simulink model "PubIfDecisionTOS_MDL"  (R2020b)
settings: configuration reference "DspaceConfig" (kept outside this file)
PostLoadFcn:
  | if any(exist('dsrtsu_mdlpostloadfcn', 'file') ~= 0), dsrtsu_mdlpostloadfcn('Execute', bdroot); end
InitFcn:
  | , if any(exist('dsmpb_private', 'file') ~= 0), dsmpb_private('dsmpb_mdlclblib', 'Init', bdroot); end,
undefined symbols (not defined in the file or in its folder): C_TOS_ACCEgoRAxletoFbumplength_m, C_TOS_ACCTargetFront_Flag, C_TOS_AEBJAPedObjDxThre_Val, C_TOS_AEBJAPedObjDyThre_Val, C_TOS_AEBJATargetSize_Val, C_TOS_AEBJAVehObjDxThre_Val, C_TOS_AEBJAVehObjDyThre_Val, C_TOS_AEBJuncPedTargetSize_Val, C_TOS_AEBLatObjDxThre_Val, C_TOS_AEBLatPedDyThre_Val, C_TOS_AEBLatTargetSize_Val, C_TOS_AEBLongTargetInEgoFront_Flag, C_TOS_axAbsGround_Parameter, C_TOS_CameraConfirmedFlag, C_TOS_CNsubjWidth, C_TOS_CurrentLaneCoreMinWidth_Val, C_TOS_CutInProb_Val_Zero, C_TOS_CutOutProb_Val_Zero, C_TOS_D2R_Val, C_TOS_DefaultValueObjectToCenterLine_dy, C_TOS_EgoCarWidth_Val, C_TOS_EgoDxRefPoint_m, C_TOS_EgoRAxletoFbumplength_m, C_TOS_HalfWidthVehicle_Con, C_TOS_HWA_CurrentLaneFlag, C_TOS_HWA_LeftLaneFlag, C_TOS_HWA_MovingDir_Vaild, C_TOS_HWA_MovState_Vaild, C_TOS_HWA_RightLaneFlag, C_TOS_LaneLineCourseErrorFront, C_TOS_LaneLineCourseErrorRear, C_TOS_MotorbikeDefaultWidth_m, C_TOS_NumberOfEffectiveTargets, C_TOS_Obj_Age_Val, C_TOS_Objdx_Constraint_Val, C_TOS_ObjectDefaultWidth_m, C_TOS_ObjInCurrentLane_Val, C_TOS_ObjInCurrentLaneValid, C_TOS_ObjInLeftLaneValid, C_TOS_ObjInRightLaneValid, C_TOS_ObjNotInCurrentLane_Val, C_TOS_ObjNotREElementType, C_TOS_ObjPredictDis_dy_ConstantVal_Zeros, C_TOS_ObjToCenterLine_ConstantVal_Zeros, C_TOS_OFMObjIDInvilad_Val, C_TOS_PIL_LatDisCons_Val_zero, C_TOS_PIL_ObjectCutInFlag_b, C_TOS_PIL_ObjectCutOutFlag_b, C_TOS_PIL_ObjLaneProb_al_Val, C_TOS_PP_ObjFusType_FC_Confirm_b, C_TOS_PP_ObjFusType_FC_FR_Confirm_b, C_TOS_PP_ObjFusType_FR_Confirm_b, C_TOS_RE_80BoolDefault_Val, C_TOS_RE_80Single181Default_Val, C_TOS_RE_80Single255Default_Val, C_TOS_RE_80Uint8Default_Val, C_TOS_RE_D2R, C_TOS_RE_D_180_Val, C_TOS_RE_InvalidObjectID_Val, C_TOS_RE_InvalidTargetChainDir_Val ... (+142)
libraries: simulink x1650, TOS_LIB x361, canfdmsglib x14
(part 28 of 69)

== system PubIfDecisionTOS_MDL/TOS_20201112/TOS_2012080320/TOS/ACC/TOS_ACCRightLane/ACC_LeftLane_Target/TOS_ACC_P3/ACC_P3_Targe ==
  ACC_P3_Index : Inport
  Object_Fus_Type : Inport  Port=2
  object_MovingState : Inport  Port=3
  PP_ObjMovingDirSignalProcessing : Inport  Port=4
  Object_HeadingAngle : Inport  Port=5
  Object_DX : Inport  Port=6
  Object_Type : Inport  Port=7
  Object_ObstacleProb : Inport  Port=8
  Object_DY : Inport  Port=9
  PP_ObjFusType_FC_FR_Confirm : Inport  Port=10
  PP_ObjFusType_FR_Confirm : Inport  Port=11
  PP_ObjFusType_FC_Confirm : Inport  Port=12
  Object_VX : Inport  Port=13
  Object_VY : Inport  Port=14
  VIE_EgoVelocity : Inport  Port=15
  SteerWheelAng : Inport  Port=16
  ACC_Target_ID_K1 : Inport  Port=17
  ACC_Target_ID_K2 : Inport  Port=18
  ACC_Target_MovState_K1 : Inport  Port=19
  ACC_Target_MovState_K2 : Inport  Port=20
  ObjectID : Inport  Port=21
  Action Port : ActionPort  ActionPortLabel=else
  ACC_P3_Targe : Subsystem
  Selector{1..3,5..13,15..16} (14 alike) : Selector  InputPortWidth=80  IndexOptions=Index vector (port)  Indices=[1 3]  OutputSizes=1
  ACC_P3_TargeConfirm : Outport
  TOS_ACC_FusionType_ObserVale : Outport  Port=2
  TOS_ACC_TrgMovDir_ObserVale : Outport  Port=3
  TOS_ACC_TargetDxConfirm_ObserVale : Outport  Port=4
  TOS_ACC_ObjType_ObserVale : Outport  Port=5
  TOS_ACC_ObstacleProb_ObserVale : Outport  Port=6
  TOS_ACC_TrgMovDirFlag_1_ObserVale : Outport  Port=7
  TOS_ACC_TrgMovDirFlag_2_ObserVale : Outport  Port=8
  TOS_ACC_TrgMovDirFlag_3_ObserVale : Outport  Port=9
  TOS_ACC_TrgMovDirFlag_4_ObserVale : Outport  Port=10
  TOS_ACC_TrgMovDirFlag_5_ObserVale : Outport  Port=11
  TOS_ACC_TrgMovDirFlag_6_ObserVale : Outport  Port=12
  wires:
  ACC_P3_Targe/12(TOS_ACC_TrgMovDirFlag_6_ObserVale) -> TOS_ACC_TrgMovDirFlag_6_ObserVale/1
  ACC_P3_Targe/11(TOS_ACC_TrgMovDirFlag_5_ObserVale) -> TOS_ACC_TrgMovDirFlag_5_ObserVale/1
  ACC_P3_Targe/1(ACC_P3_TargeConfirm) -> ACC_P3_TargeConfirm/1
  ACC_P3_Targe/10(TOS_ACC_TrgMovDirFlag_4_ObserVale) -> TOS_ACC_TrgMovDirFlag_4_ObserVale/1
  ACC_P3_Targe/2(TOS_ACC_FusionType_ObserVale) -> TOS_ACC_FusionType_ObserVale/1
  ACC_P3_Targe/9(TOS_ACC_TrgMovDirFlag_3_ObserVale) -> TOS_ACC_TrgMovDirFlag_3_ObserVale/1
  ACC_P3_Targe/3(TOS_ACC_TrgMovDir_ObserVale) -> TOS_ACC_TrgMovDir_ObserVale/1
  ACC_P3_Targe/8(TOS_ACC_TrgMovDirFlag_2_ObserVale) -> TOS_ACC_TrgMovDirFlag_2_ObserVale/1
  ACC_P3_Targe/4(TOS_ACC_TargetDxConfirm_ObserVale) -> TOS_ACC_TargetDxConfirm_ObserVale/1
  ACC_P3_Targe/7(TOS_ACC_TrgMovDirFlag_1_ObserVale) -> TOS_ACC_TrgMovDirFlag_1_ObserVale/1
  ACC_P3_Targe/5(TOS_ACC_ObjType_ObserVale) -> TOS_ACC_ObjType_ObserVale/1
  ACC_P3_Targe/6(TOS_ACC_ObstacleProb_ObserVale) -> TOS_ACC_ObstacleProb_ObserVale/1
  ACC_P3_Index/1 -> Selector16/2, Selector3/2, Selector2/2, Selector5/2, Selector6/2, Selector7/2, Selector8/2, Selector9/2, Selector10/2, Selector11/2, Selector15/2, Selector12/2, Selector13/2, Selector1/2
  Selector3/1 -> ACC_P3_Targe/20(ObjectID)
  Selector2/1 -> ACC_P3_Targe/13(Object_VY)
  Selector5/1 -> ACC_P3_Targe/12(Object_VX)
  Selector6/1 -> ACC_P3_Targe/11(PP_ObjFusType_FC_Confirm)
  Selector7/1 -> ACC_P3_Targe/10(PP_ObjFusType_FR_Confirm)
  Selector8/1 -> ACC_P3_Targe/9(PP_ObjFusType_FC_FR_Confirm)
  Selector9/1 -> ACC_P3_Targe/8(Object_DY)
  Selector10/1 -> ACC_P3_Targe/7(Object_ObstacleProb)
  Selector11/1 -> ACC_P3_Targe/6(Object_Type)
  Selector15/1 -> ACC_P3_Targe/5(Object_DX)
  Selector16/1 -> ACC_P3_Targe/4(Object_HeadingAngle)
  Selector12/1 -> ACC_P3_Targe/3(PP_ObjMovingDirSignalProcessing)
  Selector13/1 -> ACC_P3_Targe/2(object_MovingState)
  Selector1/1 -> ACC_P3_Targe/1(Object_Fus_Type)
  ObjectID/1 -> Selector3/1
  ACC_Target_MovState_K2/1 -> ACC_P3_Targe/19(ACC_Target_MovState_K2)
  ACC_Target_MovState_K1/1 -> ACC_P3_Targe/18(ACC_Target_MovState_K1)
  ACC_Target_ID_K2/1 -> ACC_P3_Targe/17(ACC_Target_ID_K2)
  ACC_Target_ID_K1/1 -> ACC_P3_Targe/16(ACC_Target_ID_K1)
  SteerWheelAng/1 -> ACC_P3_Targe/15(SteerWheelAng)
  VIE_EgoVelocity/1 -> ACC_P3_Targe/14(VIE_EgoVelocity)
  Object_VY/1 -> Selector2/1
  Object_VX/1 -> Selector5/1
  PP_ObjFusType_FC_Confirm/1 -> Selector6/1
  PP_ObjFusType_FR_Confirm/1 -> Selector7/1
  PP_ObjFusType_FC_FR_Confirm/1 -> Selector8/1
  Object_DY/1 -> Selector9/1
  Object_ObstacleProb/1 -> Selector10/1
  Object_Type/1 -> Selector11/1
  Object_DX/1 -> Selector15/1
  Object_HeadingAngle/1 -> Selector16/1
  PP_ObjMovingDirSignalProcessing/1 -> Selector12/1
  object_MovingState/1 -> Selector13/1
  Object_Fus_Type/1 -> Selector1/1

== system PubIfDecisionTOS_MDL/TOS_20201112/TOS_2012080320/TOS/ACC/TOS_ACCRightLane/ACC_LeftLane_Target/TOS_ACC_P3/ACC_P3_TargeDefault ==
  Action Port : ActionPort  ActionPortLabel=if(u1 ~= 0)
  Constant{1..6,8..13} (12 alike) : Constant  Value=0  OutDataTypeStr=boolean
  ACC_P3_TargeConfirm : Outport
  TOS_ACC_FusionType_ObserVale : Outport  Port=2
  TOS_ACC_TrgMovDir_ObserVale : Outport  Port=3
  TOS_ACC_TargetDxConfirm_ObserVale : Outport  Port=4
  TOS_ACC_ObjType_ObserVale : Outport  Port=5
  TOS_ACC_ObstacleProb_ObserVale : Outport  Port=6
  TOS_ACC_TrgMovDirFlag_1_ObserVale : Outport  Port=7
  TOS_ACC_TrgMovDirFlag_2_ObserVale : Outport  Port=8
  TOS_ACC_TrgMovDirFlag_3_ObserVale : Outport  Port=9
  TOS_ACC_TrgMovDirFlag_4_ObserVale : Outport  Port=10
  TOS_ACC_TrgMovDirFlag_5_ObserVale : Outport  Port=11
  TOS_ACC_TrgMovDirFlag_6_ObserVale : Outport  Port=12
  wires:
  Constant13/1 -> TOS_ACC_TrgMovDirFlag_6_ObserVale/1
  Constant12/1 -> TOS_ACC_TrgMovDirFlag_5_ObserVale/1
  Constant11/1 -> TOS_ACC_TrgMovDirFlag_4_ObserVale/1
  Constant10/1 -> TOS_ACC_TrgMovDirFlag_3_ObserVale/1
  Constant9/1 -> TOS_ACC_TrgMovDirFlag_2_ObserVale/1
  Constant8/1 -> TOS_ACC_TrgMovDirFlag_1_ObserVale/1
  Constant6/1 -> TOS_ACC_ObstacleProb_ObserVale/1
  Constant5/1 -> TOS_ACC_ObjType_ObserVale/1
  Constant4/1 -> TOS_ACC_TargetDxConfirm_ObserVale/1
  Constant3/1 -> TOS_ACC_TrgMovDir_ObserVale/1
  Constant1/1 -> TOS_ACC_FusionType_ObserVale/1
  Constant2/1 -> ACC_P3_TargeConfirm/1

== system PubIfDecisionTOS_MDL/TOS_20201112/TOS_2012080320/TOS/ACC/TOS_ACCRightLane/ACC_LeftLane_Target/TOS_ACC_P5/ACC_P5_Targe ==
  ACC_P5_Index : Inport
  Object_Fus_Type : Inport  Port=2
  object_MovingState : Inport  Port=3
  PP_ObjMovingDirSignalProcessing : Inport  Port=4
  Object_HeadingAngle : Inport  Port=5
  Object_DX : Inport  Port=6
  Object_Type : Inport  Port=7
  Object_ObstacleProb : Inport  Port=8
  Object_DY : Inport  Port=9
  PP_ObjFusType_FC_FR_Confirm : Inport  Port=10
  PP_ObjFusType_FR_Confirm : Inport  Port=11
  PP_ObjFusType_FC_Confirm : Inport  Port=12
  Object_VX : Inport  Port=13
  Object_VY : Inport  Port=14
  VIE_EgoVelocity : Inport  Port=15
  SteerWheelAng : Inport  Port=16
  ACC_Target_ID_K1 : Inport  Port=17
  ACC_Target_ID_K2 : Inport  Port=18
  ACC_Target_MovState_K1 : Inport  Port=19
  ACC_Target_MovState_K2 : Inport  Port=20
  ObjectID : Inport  Port=21
  Action Port : ActionPort  ActionPortLabel=else
  ACC_P5_Targe : Subsystem
  Selector{1..3,5..13,15..16} (14 alike) : Selector  InputPortWidth=80  IndexOptions=Index vector (port)  Indices=[1 3]  OutputSizes=1
  ACC_P5_TargeConfirm : Outport
  TOS_ACC_FusionType_ObserVale : Outport  Port=2
  TOS_ACC_TrgMovDir_ObserVale : Outport  Port=3
  TOS_ACC_TargetDxConfirm_ObserVale : Outport  Port=4
  TOS_ACC_ObjType_ObserVale : Outport  Port=5
  TOS_ACC_ObstacleProb_ObserVale : Outport  Port=6
  TOS_ACC_TrgMovDirFlag_1_ObserVale : Outport  Port=7
  TOS_ACC_TrgMovDirFlag_2_ObserVale : Outport  Port=8
  TOS_ACC_TrgMovDirFlag_3_ObserVale : Outport  Port=9
  TOS_ACC_TrgMovDirFlag_4_ObserVale : Outport  Port=10
  TOS_ACC_TrgMovDirFlag_5_ObserVale : Outport  Port=11
  TOS_ACC_TrgMovDirFlag_6_ObserVale : Outport  Port=12
  wires:
  Object_Fus_Type/1 -> Selector1/1
  object_MovingState/1 -> Selector13/1
  PP_ObjMovingDirSignalProcessing/1 -> Selector12/1
  Object_HeadingAngle/1 -> Selector16/1
  Object_DX/1 -> Selector15/1
  Object_Type/1 -> Selector11/1
  Object_ObstacleProb/1 -> Selector10/1
  Object_DY/1 -> Selector9/1
  PP_ObjFusType_FC_FR_Confirm/1 -> Selector8/1
  PP_ObjFusType_FR_Confirm/1 -> Selector7/1
  PP_ObjFusType_FC_Confirm/1 -> Selector6/1
  Object_VX/1 -> Selector5/1
  Object_VY/1 -> Selector2/1
  VIE_EgoVelocity/1 -> ACC_P5_Targe/14(VIE_EgoVelocity)
  SteerWheelAng/1 -> ACC_P5_Targe/15(SteerWheelAng)
  ACC_Target_ID_K1/1 -> ACC_P5_Targe/16(ACC_Target_ID_K1)
  ACC_Target_ID_K2/1 -> ACC_P5_Targe/17(ACC_Target_ID_K2)
  ACC_Target_MovState_K1/1 -> ACC_P5_Targe/18(ACC_Target_MovState_K1)
  ACC_Target_MovState_K2/1 -> ACC_P5_Targe/19(ACC_Target_MovState_K2)
  ObjectID/1 -> Selector3/1
  Selector1/1 -> ACC_P5_Targe/1(Object_Fus_Type)
  Selector13/1 -> ACC_P5_Targe/2(object_MovingState)
  Selector12/1 -> ACC_P5_Targe/3(PP_ObjMovingDirSignalProcessing)
  Selector16/1 -> ACC_P5_Targe/4(Object_HeadingAngle)
  Selector15/1 -> ACC_P5_Targe/5(Object_DX)
  Selector11/1 -> ACC_P5_Targe/6(Object_Type)
  Selector10/1 -> ACC_P5_Targe/7(Object_ObstacleProb)
  Selector9/1 -> ACC_P5_Targe/8(Object_DY)
  Selector8/1 -> ACC_P5_Targe/9(PP_ObjFusType_FC_FR_Confirm)
  Selector7/1 -> ACC_P5_Targe/10(PP_ObjFusType_FR_Confirm)
  Selector6/1 -> ACC_P5_Targe/11(PP_ObjFusType_FC_Confirm)
  Selector5/1 -> ACC_P5_Targe/12(Object_VX)
  Selector2/1 -> ACC_P5_Targe/13(Object_VY)
  Selector3/1 -> ACC_P5_Targe/20(ObjectID)
  ACC_P5_Index/1 -> Selector1/2, Selector13/2, Selector12/2, Selector15/2, Selector11/2, Selector10/2, Selector9/2, Selector8/2, Selector7/2, Selector6/2, Selector5/2, Selector2/2, Selector3/2, Selector16/2
  ACC_P5_Targe/6(TOS_ACC_ObstacleProb_ObserVale) -> TOS_ACC_ObstacleProb_ObserVale/1
  ACC_P5_Targe/5(TOS_ACC_ObjType_ObserVale) -> TOS_ACC_ObjType_ObserVale/1
  ACC_P5_Targe/7(TOS_ACC_TrgMovDirFlag_1_ObserVale) -> TOS_ACC_TrgMovDirFlag_1_ObserVale/1
  ACC_P5_Targe/4(TOS_ACC_TargetDxConfirm_ObserVale) -> TOS_ACC_TargetDxConfirm_ObserVale/1
  ACC_P5_Targe/8(TOS_ACC_TrgMovDirFlag_2_ObserVale) -> TOS_ACC_TrgMovDirFlag_2_ObserVale/1
  ACC_P5_Targe/3(TOS_ACC_TrgMovDir_ObserVale) -> TOS_ACC_TrgMovDir_ObserVale/1
  ACC_P5_Targe/9(TOS_ACC_TrgMovDirFlag_3_ObserVale) -> TOS_ACC_TrgMovDirFlag_3_ObserVale/1
  ACC_P5_Targe/2(TOS_ACC_FusionType_ObserVale) -> TOS_ACC_FusionType_ObserVale/1
  ACC_P5_Targe/10(TOS_ACC_TrgMovDirFlag_4_ObserVale) -> TOS_ACC_TrgMovDirFlag_4_ObserVale/1
  ACC_P5_Targe/1(ACC_P5_TargeConfirm) -> ACC_P5_TargeConfirm/1
  ACC_P5_Targe/11(TOS_ACC_TrgMovDirFlag_5_ObserVale) -> TOS_ACC_TrgMovDirFlag_5_ObserVale/1
  ACC_P5_Targe/12(TOS_ACC_TrgMovDirFlag_6_ObserVale) -> TOS_ACC_TrgMovDirFlag_6_ObserVale/1

== system PubIfDecisionTOS_MDL/TOS_20201112/TOS_2012080320/TOS/ACC/TOS_ACCRightLane/ACC_LeftLane_Target/TOS_ACC_P5/ACC_P5_TargeDefault ==
  Action Port : ActionPort  ActionPortLabel=if(u1 ~= 0)
  Constant{1..6,8..13} (12 alike) : Constant  Value=0  OutDataTypeStr=boolean
  ACC_P5_TargeConfirm : Outport
  TOS_ACC_FusionType_ObserVale : Outport  Port=2
  TOS_ACC_TrgMovDir_ObserVale : Outport  Port=3
  TOS_ACC_TargetDxConfirm_ObserVale : Outport  Port=4
  TOS_ACC_ObjType_ObserVale : Outport  Port=5
  TOS_ACC_ObstacleProb_ObserVale : Outport  Port=6
  TOS_ACC_TrgMovDirFlag_1_ObserVale : Outport  Port=7
  TOS_ACC_TrgMovDirFlag_2_ObserVale : Outport  Port=8
  TOS_ACC_TrgMovDirFlag_3_ObserVale : Outport  Port=9
  TOS_ACC_TrgMovDirFlag_4_ObserVale : Outport  Port=10
  TOS_ACC_TrgMovDirFlag_5_ObserVale : Outport  Port=11
  TOS_ACC_TrgMovDirFlag_6_ObserVale : Outport  Port=12
  wires:
  Constant2/1 -> ACC_P5_TargeConfirm/1
  Constant1/1 -> TOS_ACC_FusionType_ObserVale/1
  Constant3/1 -> TOS_ACC_TrgMovDir_ObserVale/1
  Constant4/1 -> TOS_ACC_TargetDxConfirm_ObserVale/1
  Constant5/1 -> TOS_ACC_ObjType_ObserVale/1
  Constant6/1 -> TOS_ACC_ObstacleProb_ObserVale/1
  Constant8/1 -> TOS_ACC_TrgMovDirFlag_1_ObserVale/1
  Constant9/1 -> TOS_ACC_TrgMovDirFlag_2_ObserVale/1
  Constant10/1 -> TOS_ACC_TrgMovDirFlag_3_ObserVale/1
  Constant11/1 -> TOS_ACC_TrgMovDirFlag_4_ObserVale/1
  Constant12/1 -> TOS_ACC_TrgMovDirFlag_5_ObserVale/1
  Constant13/1 -> TOS_ACC_TrgMovDirFlag_6_ObserVale/1

== system PubIfDecisionTOS_MDL/TOS_20201112/TOS_2012080320/TOS/ACC/TOS_ACCRightLane/ACC_Object_PreConfirm/ACC_Object_PreConfirm/ACC_Object_PreConfirm ==
  Object_ID : Inport
  PP_ObjFusType_FC_FR_Confirm : Inport  Port=2
  PP_ObjFusType_FR_Confirm : Inport  Port=3
  PP_ObjFusType_FC_Confirm : Inport  Port=4
  Obj_MovingState : Inport  Port=5
  Obj_Dx : Inport  Port=6
  Object_ObstacleProb : Inport  Port=7
  Object_DY : Inport  Port=8
  Object_ObjType : Inport  Port=9
  ACC_Target_ID_K1 : Inport  Port=10
  ACC_Target_Dx_K1 : Inport  Port=11
  Action Port : ActionPort  ActionPortLabel=else
  " " : Subsystem
  Bus Creator : BusCreator  Inputs=11
  Bus Selector1 : BusSelector  OutputSignals=PP_ObjFusType_FC_Confirm,Obj_MovingState
  Bus Selector2 : BusSelector  OutputSignals=PP_ObjFusType_FC_FR_Confirm,PP_ObjFusType_FC_Confirm,PP_ObjFusType_FR_Confirm
  Bus Selector4 : BusSelector  OutputSignals=Object_ObjType
  Constant1 : Constant  OutDataTypeStr=boolean
  Logical Operator1 : Logic  Inputs=4  AllPortsSameDT=off  OutDataTypeStr=boolean
  Subsystem : Subsystem
  Subsystem1 : Subsystem
  TOS_ACC_DyConfirm : Subsystem
  Terminator : Terminator
  TOS_ACC_TargetPre_Confirm_FiltFlag : Outport
  TOS_ACC_TargetPre_FusionTypeFlag_ObserVale : Outport  Port=2
  TOS_ACC_TargetPre_PassedbyTarget_ObserVale : Outport  Port=3
  TOS_ACC_TargetPre_ObjType_ObserVale : Outport  Port=4
  TOS_ACC_DyConfirm_ObserVale : Outport  Port=5
  wires:
  TOS_ACC_DyConfirm/1(TOS_ACC_TargetPre_DyConfirm) -> Terminator/1
  Bus Creator/1 -> Bus Selector2/1, Bus Selector1/1, Bus Selector4/1, TOS_ACC_DyConfirm/1(TOS_ACC_Dy)
  Logical Operator1/1 -> TOS_ACC_TargetPre_Confirm_FiltFlag/1
  [TOS_ACC_DyConfirm_ObserVale] -> TOS_ACC_DyConfirm_ObserVale/1
  Constant1/1 -> [TOS_ACC_DyConfirm_ObserVale], Logical Operator1/4
  [TOS_ACC_TargetPre_ObjType_ObserVale] -> TOS_ACC_TargetPre_ObjType_ObserVale/1
  [TOS_ACC_TargetPre_PassedbyTarget_Flag_ObserVale] -> TOS_ACC_TargetPre_PassedbyTarget_ObserVale/1
  [TOS_ACC_TargetPre_FusionTypeFlag_ObserVale] -> TOS_ACC_TargetPre_FusionTypeFlag_ObserVale/1
  Object_ObjType/1 -> Bus Creator/9  "Object_ObjType"
  " "/1(TOS_ACC_TargetPre_ObjType) -> [TOS_ACC_TargetPre_ObjType_ObserVale], Logical Operator1/3
  Bus Selector4/1 -> " "/1(Object_Type)  "<Object_ObjType>"
  Obj_Dx/1 -> Bus Creator/6  "Obj_Dx"
  Object_ObstacleProb/1 -> Bus Creator/7  "Object_ObstacleProb"
  Obj_MovingState/1 -> Bus Creator/5  "Obj_MovingState"
  ACC_Target_Dx_K1/1 -> Bus Creator/11  "ACC_Target_Dx_K1"
  Bus Selector1/2 -> Subsystem1/2(Obj_MovingState)  "<Obj_MovingState>"
  Object_DY/1 -> Bus Creator/8  "Object_DY"
  ACC_Target_ID_K1/1 -> Bus Creator/10  "ACC_Target_ID_K1"
  PP_ObjFusType_FC_FR_Confirm/1 -> Bus Creator/2  "PP_ObjFusType_FC_FR_Confirm"
  Bus Selector2/2 -> Subsystem/2(PP_ObjFusType_FR_Confirm)  "<PP_ObjFusType_FC_Confirm>"
  Bus Selector1/1 -> Subsystem1/1(PP_ObjFusType_FC_Confirm)  "<PP_ObjFusType_FC_Confirm>"
  Bus Selector2/3 -> Subsystem/3(PP_ObjFusType_FC_Confirm)  "<PP_ObjFusType_FR_Confirm>"
  Bus Selector2/1 -> Subsystem/1(PP_ObjFusType_FC_FR_Confirm)  "<PP_ObjFusType_FC_FR_Confirm>"
  PP_ObjFusType_FC_Confirm/1 -> Bus Creator/4  "PP_ObjFusType_FC_Confirm"
  Object_ID/1 -> Bus Creator/1  "Object_ID"
  PP_ObjFusType_FR_Confirm/1 -> Bus Creator/3  "PP_ObjFusType_FR_Confirm"
  Subsystem1/1(TOS_ACC_TargetPre_ObjectPassedbyTarget_Flag) -> Logical Operator1/2, [TOS_ACC_TargetPre_PassedbyTarget_Flag_ObserVale]
  Subsystem/1(TOS_ACC_TargetPre_TargetFusionTypeFlag) -> Logical Operator1/1, [TOS_ACC_TargetPre_FusionTypeFlag_ObserVale]

== system PubIfDecisionTOS_MDL/TOS_20201112/TOS_2012080320/TOS/ACC/TOS_ACCRightLane/ACC_Object_PreConfirm/ACC_Object_PreConfirm/ACC_Object_PreConfirmDefault ==
  Action Port : ActionPort  ActionPortLabel=if(u1 ~= 0)
  Constant{2,5..6,8,10} (5 alike) : Constant  Value=0  OutDataTypeStr=boolean
  TOS_ACC_TargetPre_Confirm_FiltFlag : Outport
  TOS_ACC_TargetPre_FusionTypeFlag_ObserVale : Outport  Port=2
  TOS_ACC_TargetPre_PassedbyTarget_ObserVale : Outport  Port=3
  TOS_ACC_TargetPre_ObjType_ObserVale : Outport  Port=4
  TOS_ACC_DyConfirm_ObserVale : Outport  Port=5
  wires:
  Constant10/1 -> TOS_ACC_DyConfirm_ObserVale/1
  Constant8/1 -> TOS_ACC_TargetPre_ObjType_ObserVale/1
  Constant6/1 -> TOS_ACC_TargetPre_PassedbyTarget_ObserVale/1
  Constant5/1 -> TOS_ACC_TargetPre_FusionTypeFlag_ObserVale/1
  Constant2/1 -> TOS_ACC_TargetPre_Confirm_FiltFlag/1

== system PubIfDecisionTOS_MDL/TOS_20201112/TOS_2012080320/TOS/AEB/TOS_AEBJunct1105/AEBJunc_Object_Condition/AEBJA_TargetCondition/TOS_AEBJunc_TargetsCondition ==
  Object_ID : Inport
  PP_ObjFusType_FC_FR_Confirm : Inport  Port=2
  PP_ObjFusType_FR_Confirm : Inport  Port=3
  ObjectType : Inport  Port=4
  Object_Dx : Inport  Port=5
  Object_Dy : Inport  Port=6
  PP_ObjMovingDirSignalProcessing : Inport  Port=7
  Object_HeadingAngle : Inport  Port=8
  Object_VX : Inport  Port=9
  Object_VY : Inport  Port=10
  VIE_EgoVelocity : Inport  Port=11
  psiDtOpt : Inport  Port=12
  axvRefMs2 : Inport  Port=13
  Object_MovingState : Inport  Port=14
  AEBJunc_Target_ObjectID_K1 : Inport  Port=15
  AEBJunc_Target_ObjectType_K1 : Inport  Port=16
  Action Port : ActionPort
  AEBJunc_PedTargetCondition : Subsystem
  AEBJunc_VehTargetCondition : Subsystem
  Bus Creator : BusCreator  Inputs=16
  Bus Selector : BusSelector  OutputSignals=Object_ID,PP_ObjFusType_FC_FR_Confirm,PP_ObjFusType_FR_Confirm,ObjectType,Object_Dx,Object_Dy,PP_ObjMovingDirSignalProcessing,Object_HeadingAngle,Object_VX,Object_VY,VIE_EgoVelocity,psiDtOpt,axvRefMs2,AEBJunc_Target_ObjectID_K1,AEBJunc_Target_ObjectType_K1
  Bus Selector1 : BusSelector  OutputSignals=Object_ID,PP_ObjFusType_FC_FR_Confirm,PP_ObjFusType_FR_Confirm,ObjectType,Object_Dx,Object_Dy,PP_ObjMovingDirSignalProcessing,Object_HeadingAngle,Object_VX,Object_VY,VIE_EgoVelocity,psiDtOpt,axvRefMs2,AEBJunc_Target_ObjectID_K1,AEBJunc_Target_ObjectType_K1,Object_MovingState
  TOS_AEBJunc_PedTargetsDx : Outport
  TOS_AEBJunc_VehTargetsDx : Outport  Port=2
  AEBJunc_PedTargetFusionType_observal : Outport  Port=3
  AEBJunc_PedTargetObjectType_observal : Outport  Port=4
  AEBJunc_PedTargetDXDY_observal : Outport  Port=5
  AEBJunc_PedTargetMovDir_observal : Outport  Port=6
  AEBJunc_VehTargetFusionType_observal : Outport  Port=7
  AEBJunc_VehTargetObjectType_observal : Outport  Port=8
  AEBJunc_VehTargetDXDY_observal : Outport  Port=9
  AEBJunc_VehTargetMovDir_observal : Outport  Port=10
  AEBJunc_VehTargetMovState_observal : Outport  Port=11
  wires:
  AEBJunc_PedTargetCondition/1(TOS_AEBJunc_PedTargetsDx) -> TOS_AEBJunc_PedTargetsDx/1
  AEBJunc_PedTargetCondition/2(AEBJunc_PedTargetFusionType_observal) -> AEBJunc_PedTargetFusionType_observal/1
  AEBJunc_PedTargetCondition/3(AEBJunc_PedTargetObjectType_observal) -> AEBJunc_PedTargetObjectType_observal/1
  AEBJunc_PedTargetCondition/4(AEBJunc_PedTargetDXDY_observal) -> AEBJunc_PedTargetDXDY_observal/1
  AEBJunc_PedTargetCondition/5(AEBJunc_PedTargetMovDir_observal) -> AEBJunc_PedTargetMovDir_observal/1
  Object_ID/1 -> Bus Creator/1  "Object_ID"
  PP_ObjFusType_FC_FR_Confirm/1 -> Bus Creator/2  "PP_ObjFusType_FC_FR_Confirm"
  PP_ObjFusType_FR_Confirm/1 -> Bus Creator/3  "PP_ObjFusType_FR_Confirm"
  ObjectType/1 -> Bus Creator/4  "ObjectType"
  Object_Dx/1 -> Bus Creator/5  "Object_Dx"
  Object_Dy/1 -> Bus Creator/6  "Object_Dy"
  PP_ObjMovingDirSignalProcessing/1 -> Bus Creator/7  "PP_ObjMovingDirSignalProcessing"
  Object_HeadingAngle/1 -> Bus Creator/8  "Object_HeadingAngle"
  Object_VX/1 -> Bus Creator/9  "Object_VX"
  Object_VY/1 -> Bus Creator/10  "Object_VY"
  VIE_EgoVelocity/1 -> Bus Creator/11  "VIE_EgoVelocity"
  psiDtOpt/1 -> Bus Creator/12  "psiDtOpt"
  axvRefMs2/1 -> Bus Creator/13  "axvRefMs2"
  AEBJunc_Target_ObjectID_K1/1 -> Bus Creator/15  "AEBJunc_Target_ObjectID_K1"
  AEBJunc_Target_ObjectType_K1/1 -> Bus Creator/16  "AEBJunc_Target_ObjectType_K1"
  Bus Creator/1 -> Bus Selector1/1, Bus Selector/1
  Bus Selector/1 -> AEBJunc_PedTargetCondition/1(Object_ID)  "<Object_ID>"
  Bus Selector/2 -> AEBJunc_PedTargetCondition/2(PP_ObjFusType_FC_FR_Confirm)  "<PP_ObjFusType_FC_FR_Confirm>"
  Bus Selector/3 -> AEBJunc_PedTargetCondition/3(PP_ObjFusType_FR_Confirm)  "<PP_ObjFusType_FR_Confirm>"
  Bus Selector/4 -> AEBJunc_PedTargetCondition/4(ObjectType)  "<ObjectType>"
  Bus Selector/5 -> AEBJunc_PedTargetCondition/5(Object_Dx)  "<Object_Dx>"
  Bus Selector/6 -> AEBJunc_PedTargetCondition/6(Object_Dy)  "<Object_Dy>"
  Bus Selector/7 -> AEBJunc_PedTargetCondition/7(PP_ObjMovingDirSignalProcessing)  "<PP_ObjMovingDirSignalProcessing>"
  Bus Selector/8 -> AEBJunc_PedTargetCondition/8(Object_HeadingAngle)  "<Object_HeadingAngle>"
  Bus Selector/9 -> AEBJunc_PedTargetCondition/9(Object_VX)  "<Object_VX>"
  Bus Selector/10 -> AEBJunc_PedTargetCondition/10(Object_VY)  "<Object_VY>"
  Bus Selector/11 -> AEBJunc_PedTargetCondition/11(VIE_EgoVelocity)  "<VIE_EgoVelocity>"
  Bus Selector/12 -> AEBJunc_PedTargetCondition/12(psiDtOpt)  "<psiDtOpt>"
  Bus Selector/13 -> AEBJunc_PedTargetCondition/13(axvRefMs2)  "<axvRefMs2>"
  Bus Selector/14 -> AEBJunc_PedTargetCondition/14(AEBJunc_PedTarget_ObjectID_K1)  "<AEBJunc_Target_ObjectID_K1>"
  Bus Selector/15 -> AEBJunc_PedTargetCondition/15(AEBJunc_Target_ObjectType_K1)  "<AEBJunc_Target_ObjectType_K1>"
  Bus Selector1/15 -> AEBJunc_VehTargetCondition/15(AEBJunc_Target_ObjectType_K1)  "<AEBJunc_Target_ObjectType_K1>"
  Bus Selector1/14 -> AEBJunc_VehTargetCondition/14(AEBJunc_VehTarget_ObjectID_K1)  "<AEBJunc_Target_ObjectID_K1>"
  Bus Selector1/13 -> AEBJunc_VehTargetCondition/13(axvRefMs2)  "<axvRefMs2>"
  Bus Selector1/12 -> AEBJunc_VehTargetCondition/12(psiDtOpt)  "<psiDtOpt>"
  Bus Selector1/11 -> AEBJunc_VehTargetCondition/11(VIE_EgoVelocity)  "<VIE_EgoVelocity>"
  Bus Selector1/10 -> AEBJunc_VehTargetCondition/10(Object_VY)  "<Object_VY>"
  Bus Selector1/9 -> AEBJunc_VehTargetCondition/9(Object_VX)  "<Object_VX>"
  Bus Selector1/8 -> AEBJunc_VehTargetCondition/8(Object_HeadingAngle)  "<Object_HeadingAngle>"
  Bus Selector1/7 -> AEBJunc_VehTargetCondition/7(PP_ObjMovingDirSignalProcessing)  "<PP_ObjMovingDirSignalProcessing>"
  Bus Selector1/6 -> AEBJunc_VehTargetCondition/6(Object_Dy)  "<Object_Dy>"
  Bus Selector1/5 -> AEBJunc_VehTargetCondition/5(Object_Dx)  "<Object_Dx>"
  Bus Selector1/4 -> AEBJunc_VehTargetCondition/4(ObjectType)  "<ObjectType>"
  Bus Selector1/3 -> AEBJunc_VehTargetCondition/3(PP_ObjFusType_FR_Confirm)  "<PP_ObjFusType_FR_Confirm>"
  Bus Selector1/2 -> AEBJunc_VehTargetCondition/2(PP_ObjFusType_FC_FR_Confirm)  "<PP_ObjFusType_FC_FR_Confirm>"
  Bus Selector1/1 -> AEBJunc_VehTargetCondition/1(Object_ID)  "<Object_ID>"
  AEBJunc_VehTargetCondition/5(AEBJunc_VehTargetMovDir_observal) -> AEBJunc_VehTargetMovDir_observal/1
  AEBJunc_VehTargetCondition/4(AEBJunc_VehTargetDXDY_observal) -> AEBJunc_VehTargetDXDY_observal/1
  AEBJunc_VehTargetCondition/3(AEBJunc_VehTargetObjectType_observal) -> AEBJunc_VehTargetObjectType_observal/1
  AEBJunc_VehTargetCondition/2(AEBJunc_VehTargetFusionType_observal) -> AEBJunc_VehTargetFusionType_observal/1
  AEBJunc_VehTargetCondition/1(TOS_AEBJunc_VehTargetsDx) -> TOS_AEBJunc_VehTargetsDx/1
  Object_MovingState/1 -> Bus Creator/14  "Object_MovingState"
  Bus Selector1/16 -> AEBJunc_VehTargetCondition/16(Object_MovingState)  "<Object_MovingState>"
  AEBJunc_VehTargetCondition/6(AEBJunc_VehTargetMovState_observal) -> AEBJunc_VehTargetMovState_observal/1

== system PubIfDecisionTOS_MDL/TOS_20201112/TOS_2012080320/TOS/AEB/TOS_AEBJunct1105/AEBJunc_Object_Condition/AEBJA_TargetCondition/TOS_AEBJunc_TargetsConditionDefault ==
  Action Port : ActionPort
  Constant{1,3..5,7..11} (9 alike) : Constant  Value=0  OutDataTypeStr=boolean
  Constant2 : Constant  Value=255  OutDataTypeStr=single
  Constant6 : Constant  Value=255  OutDataTypeStr=single
  TOS_AEBJunc_PedTargetsDx : Outport
  TOS_AEBJunc_VehTargetsDx : Outport  Port=2
  AEBJunc_PedTargetFusionType_observal : Outport  Port=3
  AEBJunc_PedTargetObjectType_observal : Outport  Port=4
  AEBJunc_PedTargetDXDY_observal : Outport  Port=5
  AEBJunc_PedTargetMovDir_observal : Outport  Port=6
  AEBJunc_VehTargetFusionType_observal : Outport  Port=7
  AEBJunc_VehTargetObjectType_observal : Outport  Port=8
  AEBJunc_VehTargetDXDY_observal : Outport  Port=9
  AEBJunc_VehTargetMovDir_observal : Outport  Port=10
  AEBJunc_VehTargetMovState_observal : Outport  Port=11
  wires:
  Constant2/1 -> TOS_AEBJunc_PedTargetsDx/1
  Constant3/1 -> AEBJunc_PedTargetObjectType_observal/1
  Constant1/1 -> AEBJunc_PedTargetFusionType_observal/1
  Constant4/1 -> AEBJunc_PedTargetDXDY_observal/1
  Constant5/1 -> AEBJunc_PedTargetMovDir_observal/1
  Constant6/1 -> TOS_AEBJunc_VehTargetsDx/1
  Constant10/1 -> AEBJunc_VehTargetMovDir_observal/1
  Constant9/1 -> AEBJunc_VehTargetDXDY_observal/1
  Constant7/1 -> AEBJunc_VehTargetFusionType_observal/1
  Constant8/1 -> AEBJunc_VehTargetObjectType_observal/1
  Constant11/1 -> AEBJunc_VehTargetMovState_observal/1

== system PubIfDecisionTOS_MDL/TOS_20201112/TOS_2012080320/TOS/AEB/TOS_AEBJunct1105/AEBJunc_Object_Condition1/AEBJA_TargetCondition/TOS_AEBJunc_TargetsCondition ==
  Object_ID : Inport
  PP_ObjFusType_FC_FR_Confirm : Inport  Port=2
  PP_ObjFusType_FR_Confirm : Inport  Port=3
  ObjectType : Inport  Port=4
  Object_Dx : Inport  Port=5
  Object_Dy : Inport  Port=6
  PP_ObjMovingDirSignalProcessing : Inport  Port=7
  Object_HeadingAngle : Inport  Port=8
  Object_VX : Inport  Port=9
  Object_VY : Inport  Port=10
  VIE_EgoVelocity : Inport  Port=11
  psiDtOpt : Inport  Port=12
  axvRefMs2 : Inport  Port=13
  Object_MovingState : Inport  Port=14
  AEBJunc_Target_ObjectID_K1 : Inport  Port=15
  AEBJunc_Target_ObjectType_K1 : Inport  Port=16
  Action Port : ActionPort
  AEBJunc_PedTargetCondition : Subsystem
  AEBJunc_VehTargetCondition : Subsystem
  Bus Creator : BusCreator  Inputs=16
  Bus Selector : BusSelector  OutputSignals=Object_ID,PP_ObjFusType_FC_FR_Confirm,PP_ObjFusType_FR_Confirm,ObjectType,Object_Dx,Object_Dy,PP_ObjMovingDirSignalProcessing,Object_HeadingAngle,Object_VX,Object_VY,VIE_EgoVelocity,psiDtOpt,axvRefMs2,AEBJunc_Target_ObjectID_K1,AEBJunc_Target_ObjectType_K1
  Bus Selector1 : BusSelector  OutputSignals=Object_ID,PP_ObjFusType_FC_FR_Confirm,PP_ObjFusType_FR_Confirm,ObjectType,Object_Dx,Object_Dy,PP_ObjMovingDirSignalProcessing,Object_HeadingAngle,Object_VX,Object_VY,VIE_EgoVelocity,psiDtOpt,axvRefMs2,AEBJunc_Target_ObjectID_K1,AEBJunc_Target_ObjectType_K1,Object_MovingState
  TOS_AEBJunc_PedTargetsDx : Outport
  TOS_AEBJunc_VehTargetsDx : Outport  Port=2
  AEBJunc_PedTargetFusionType_observal : Outport  Port=3
  AEBJunc_PedTargetObjectType_observal : Outport  Port=4
  AEBJunc_PedTargetDXDY_observal : Outport  Port=5
  AEBJunc_PedTargetMovDir_observal : Outport  Port=6
  AEBJunc_VehTargetFusionType_observal : Outport  Port=7
  AEBJunc_VehTargetObjectType_observal : Outport  Port=8
  AEBJunc_VehTargetDXDY_observal : Outport  Port=9
  AEBJunc_VehTargetMovDir_observal : Outport  Port=10
  AEBJunc_VehTargetMovState_observal : Outport  Port=11
  wires:
  AEBJunc_VehTargetCondition/6(AEBJunc_VehTargetMovState_observal) -> AEBJunc_VehTargetMovState_observal/1
  Bus Selector1/16 -> AEBJunc_VehTargetCondition/16(Object_MovingState)  "<Object_MovingState>"
  Object_MovingState/1 -> Bus Creator/14  "Object_MovingState"
  AEBJunc_VehTargetCondition/1(TOS_AEBJunc_VehTargetsDx) -> TOS_AEBJunc_VehTargetsDx/1
  AEBJunc_VehTargetCondition/2(AEBJunc_VehTargetFusionType_observal) -> AEBJunc_VehTargetFusionType_observal/1
  AEBJunc_VehTargetCondition/3(AEBJunc_VehTargetObjectType_observal) -> AEBJunc_VehTargetObjectType_observal/1
  AEBJunc_VehTargetCondition/4(AEBJunc_VehTargetDXDY_observal) -> AEBJunc_VehTargetDXDY_observal/1
  AEBJunc_VehTargetCondition/5(AEBJunc_VehTargetMovDir_observal) -> AEBJunc_VehTargetMovDir_observal/1
  Bus Selector1/1 -> AEBJunc_VehTargetCondition/1(Object_ID)  "<Object_ID>"
  Bus Selector1/2 -> AEBJunc_VehTargetCondition/2(PP_ObjFusType_FC_FR_Confirm)  "<PP_ObjFusType_FC_FR_Confirm>"
  Bus Selector1/3 -> AEBJunc_VehTargetCondition/3(PP_ObjFusType_FR_Confirm)  "<PP_ObjFusType_FR_Confirm>"
  Bus Selector1/4 -> AEBJunc_VehTargetCondition/4(ObjectType)  "<ObjectType>"
  Bus Selector1/5 -> AEBJunc_VehTargetCondition/5(Object_Dx)  "<Object_Dx>"
  Bus Selector1/6 -> AEBJunc_VehTargetCondition/6(Object_Dy)  "<Object_Dy>"
  Bus Selector1/7 -> AEBJunc_VehTargetCondition/7(PP_ObjMovingDirSignalProcessing)  "<PP_ObjMovingDirSignalProcessing>"
  Bus Selector1/8 -> AEBJunc_VehTargetCondition/8(Object_HeadingAngle)  "<Object_HeadingAngle>"
  Bus Selector1/9 -> AEBJunc_VehTargetCondition/9(Object_VX)  "<Object_VX>"
  Bus Selector1/10 -> AEBJunc_VehTargetCondition/10(Object_VY)  "<Object_VY>"
  Bus Selector1/11 -> AEBJunc_VehTargetCondition/11(VIE_EgoVelocity)  "<VIE_EgoVelocity>"
  Bus Selector1/12 -> AEBJunc_VehTargetCondition/12(psiDtOpt)  "<psiDtOpt>"
  Bus Selector1/13 -> AEBJunc_VehTargetCondition/13(axvRefMs2)  "<axvRefMs2>"
  Bus Selector1/14 -> AEBJunc_VehTargetCondition/14(AEBJunc_VehTarget_ObjectID_K1)  "<AEBJunc_Target_ObjectID_K1>"
  Bus Selector1/15 -> AEBJunc_VehTargetCondition/15(AEBJunc_Target_ObjectType_K1)  "<AEBJunc_Target_ObjectType_K1>"
  Bus Selector/15 -> AEBJunc_PedTargetCondition/15(AEBJunc_Target_ObjectType_K1)  "<AEBJunc_Target_ObjectType_K1>"
  Bus Selector/14 -> AEBJunc_PedTargetCondition/14(AEBJunc_PedTarget_ObjectID_K1)  "<AEBJunc_Target_ObjectID_K1>"
  Bus Selector/13 -> AEBJunc_PedTargetCondition/13(axvRefMs2)  "<axvRefMs2>"
  Bus Selector/12 -> AEBJunc_PedTargetCondition/12(psiDtOpt)  "<psiDtOpt>"
  Bus Selector/11 -> AEBJunc_PedTargetCondition/11(VIE_EgoVelocity)  "<VIE_EgoVelocity>"
  Bus Selector/10 -> AEBJunc_PedTargetCondition/10(Object_VY)  "<Object_VY>"
  Bus Selector/9 -> AEBJunc_PedTargetCondition/9(Object_VX)  "<Object_VX>"
  Bus Selector/8 -> AEBJunc_PedTargetCondition/8(Object_HeadingAngle)  "<Object_HeadingAngle>"
  Bus Selector/7 -> AEBJunc_PedTargetCondition/7(PP_ObjMovingDirSignalProcessing)  "<PP_ObjMovingDirSignalProcessing>"
  Bus Selector/6 -> AEBJunc_PedTargetCondition/6(Object_Dy)  "<Object_Dy>"
  Bus Selector/5 -> AEBJunc_PedTargetCondition/5(Object_Dx)  "<Object_Dx>"
  Bus Selector/4 -> AEBJunc_PedTargetCondition/4(ObjectType)  "<ObjectType>"
  Bus Selector/3 -> AEBJunc_PedTargetCondition/3(PP_ObjFusType_FR_Confirm)  "<PP_ObjFusType_FR_Confirm>"
  Bus Selector/2 -> AEBJunc_PedTargetCondition/2(PP_ObjFusType_FC_FR_Confirm)  "<PP_ObjFusType_FC_FR_Confirm>"
  Bus Selector/1 -> AEBJunc_PedTargetCondition/1(Object_ID)  "<Object_ID>"
  Bus Creator/1 -> Bus Selector/1, Bus Selector1/1
  AEBJunc_Target_ObjectType_K1/1 -> Bus Creator/16  "AEBJunc_Target_ObjectType_K1"
  AEBJunc_Target_ObjectID_K1/1 -> Bus Creator/15  "AEBJunc_Target_ObjectID_K1"
  axvRefMs2/1 -> Bus Creator/13  "axvRefMs2"
  psiDtOpt/1 -> Bus Creator/12  "psiDtOpt"
  VIE_EgoVelocity/1 -> Bus Creator/11  "VIE_EgoVelocity"
  Object_VY/1 -> Bus Creator/10  "Object_VY"
  Object_VX/1 -> Bus Creator/9  "Object_VX"
  Object_HeadingAngle/1 -> Bus Creator/8  "Object_HeadingAngle"
  PP_ObjMovingDirSignalProcessing/1 -> Bus Creator/7  "PP_ObjMovingDirSignalProcessing"
  Object_Dy/1 -> Bus Creator/6  "Object_Dy"
  Object_Dx/1 -> Bus Creator/5  "Object_Dx"
  ObjectType/1 -> Bus Creator/4  "ObjectType"
  PP_ObjFusType_FR_Confirm/1 -> Bus Creator/3  "PP_ObjFusType_FR_Confirm"
  PP_ObjFusType_FC_FR_Confirm/1 -> Bus Creator/2  "PP_ObjFusType_FC_FR_Confirm"
  Object_ID/1 -> Bus Creator/1  "Object_ID"
  AEBJunc_PedTargetCondition/5(AEBJunc_PedTargetMovDir_observal) -> AEBJunc_PedTargetMovDir_observal/1
  AEBJunc_PedTargetCondition/4(AEBJunc_PedTargetDXDY_observal) -> AEBJunc_PedTargetDXDY_observal/1
  AEBJunc_PedTargetCondition/3(AEBJunc_PedTargetObjectType_observal) -> AEBJunc_PedTargetObjectType_observal/1
  AEBJunc_PedTargetCondition/2(AEBJunc_PedTargetFusionType_observal) -> AEBJunc_PedTargetFusionType_observal/1
  AEBJunc_PedTargetCondition/1(TOS_AEBJunc_PedTargetsDx) -> TOS_AEBJunc_PedTargetsDx/1

== system PubIfDecisionTOS_MDL/TOS_20201112/TOS_2012080320/TOS/AEB/TOS_AEBJunct1105/AEBJunc_Object_Condition1/AEBJA_TargetCondition/TOS_AEBJunc_TargetsConditionDefault ==
  Action Port : ActionPort
  Constant{1,3..5,7..11} (9 alike) : Constant  Value=0  OutDataTypeStr=boolean
  Constant2 : Constant  Value=255  OutDataTypeStr=single
  Constant6 : Constant  Value=255  OutDataTypeStr=single
  TOS_AEBJunc_PedTargetsDx : Outport
  TOS_AEBJunc_VehTargetsDx : Outport  Port=2
  AEBJunc_PedTargetFusionType_observal : Outport  Port=3
  AEBJunc_PedTargetObjectType_observal : Outport  Port=4
  AEBJunc_PedTargetDXDY_observal : Outport  Port=5
  AEBJunc_PedTargetMovDir_observal : Outport  Port=6
  AEBJunc_VehTargetFusionType_observal : Outport  Port=7
  AEBJunc_VehTargetObjectType_observal : Outport  Port=8
  AEBJunc_VehTargetDXDY_observal : Outport  Port=9
  AEBJunc_VehTargetMovDir_observal : Outport  Port=10
  AEBJunc_VehTargetMovState_observal : Outport  Port=11
  wires:
  Constant11/1 -> AEBJunc_VehTargetMovState_observal/1
  Constant8/1 -> AEBJunc_VehTargetObjectType_observal/1
  Constant7/1 -> AEBJunc_VehTargetFusionType_observal/1
  Constant9/1 -> AEBJunc_VehTargetDXDY_observal/1
  Constant10/1 -> AEBJunc_VehTargetMovDir_observal/1
  Constant6/1 -> TOS_AEBJunc_VehTargetsDx/1
  Constant5/1 -> AEBJunc_PedTargetMovDir_observal/1
  Constant4/1 -> AEBJunc_PedTargetDXDY_observal/1
  Constant1/1 -> AEBJunc_PedTargetFusionType_observal/1
  Constant3/1 -> AEBJunc_PedTargetObjectType_observal/1
  Constant2/1 -> TOS_AEBJunc_PedTargetsDx/1

== system PubIfDecisionTOS_MDL/TOS_20201112/TOS_2012080320/TOS/AEB/TOS_AEBJunct1105/AEBJunctionTargetInfor/AEBJuncTargetObjectType/AEBJuncTargetObjectType ==
  TOS_AEBJuncTrg_Index : Inport  OutDataTypeStr=uint8
  OFM_SignalVerification : Inport  Port=2
  AEBJunc_Target_ObjectID_K1 : Inport  Port=3
  AEBJunc_Target_ObjectType_K1 : Inport  Port=4
  Action Port : ActionPort
  Bus Selector1 : BusSelector  OutputSignals=Object_Type,Object_ID
  Data Type Conversion : DataTypeConversion  OutDataTypeStr=Enum: OFM_OBJ_TYPE_E
  Data Type Conversion1 : DataTypeConversion  OutDataTypeStr=uint8
  Data Type Conversion2 : DataTypeConversion  OutDataTypeStr=Enum: OFM_OBJ_TYPE_E
  Selector : Selector  InputPortWidth=80  IndexOptions=Index vector (port)  Indices=[1 3]  OutputSizes=1
  Selector1 : Selector  InputPortWidth=80  IndexOptions=Index vector (port)  Indices=[1 3]  OutputSizes=1
  TOS_AEBJunc_TargetObjectType : Stateflow chart  TreatAsAtomicUnit=on
  AEBLat_TargetObjectType : Outport
  wires:
  TOS_AEBJuncTrg_Index/1 -> Selector1/2, Selector/2
  Data Type Conversion/1 -> TOS_AEBJunc_TargetObjectType/1(ObjectType)  "Object_Type"
  Selector/1 -> Data Type Conversion/1
  OFM_SignalVerification/1 -> Bus Selector1/1
  Bus Selector1/1 -> Selector/1  "<Object_Type>"
  Data Type Conversion1/1 -> AEBLat_TargetObjectType/1
  AEBJunc_Target_ObjectType_K1/1 -> Data Type Conversion2/1
  Selector1/1 -> TOS_AEBJunc_TargetObjectType/2(Object_ID)  "Object_ID"
  Data Type Conversion2/1 -> TOS_AEBJunc_TargetObjectType/3(AEBJunc_Target_ObjectType_K1)  "AEBJunc_Target_ObjectType_K1"
  AEBJunc_Target_ObjectID_K1/1 -> TOS_AEBJunc_TargetObjectType/4(AEBJunc_Target_ObjectID_K1)  "AEBJunc_Target_ObjectID_K1"
  TOS_AEBJunc_TargetObjectType/1(AEBJunc_TargetObjectType) -> Data Type Conversion1/1  "AEBJunc_TargetObjectType"
  Bus Selector1/2 -> Selector1/1  "<Object_ID>"

== system PubIfDecisionTOS_MDL/TOS_20201112/TOS_2012080320/TOS/AEB/TOS_AEBJunct1105/AEBJunctionTargetInfor/AEBJuncTargetObjectType/AEBJuncTargetObjectTypeDefault ==
  Action Port : ActionPort
  Constant : Constant  Value=0  OutDataTypeStr=uint8
  TOS_AEBJuncTargetObjectType : Outport
  wires:
  Constant/1 -> TOS_AEBJuncTargetObjectType/1

== system PubIfDecisionTOS_MDL/TOS_20201112/TOS_2012080320/TOS/AEB/TOS_AEBJunct_20201208/AEBJunc_Object_Condition/AEBJA_TargetCondition/TOS_AEBJunc_TargetsCondition ==
  Object_ID : Inport
  PP_ObjFusType_FC_FR_Confirm : Inport  Port=2
  PP_ObjFusType_FR_Confirm : Inport  Port=3
  ObjectType : Inport  Port=4
  Object_Dx : Inport  Port=5
  Object_Dy : Inport  Port=6
  PP_ObjMovingDirSignalProcessing : Inport  Port=7
  Object_HeadingAngle : Inport  Port=8
  Object_VX : Inport  Port=9
  Object_VY : Inport  Port=10
  VIE_EgoVelocity : Inport  Port=11
  psiDtOpt : Inport  Port=12
  axvRefMs2 : Inport  Port=13
  Object_MovingState : Inport  Port=14
  AEBJunc_Target_ObjectID_K1 : Inport  Port=15
  AEBJunc_Target_ObjectType_K1 : Inport  Port=16
  Action Port : ActionPort  ActionPortLabel=else
  AEBJunc_PedTargetCondition : Subsystem
  AEBJunc_VehTargetCondition : Subsystem
  Bus Creator : BusCreator  Inputs=16
  Bus Selector : BusSelector  OutputSignals=Object_ID,PP_ObjFusType_FC_FR_Confirm,PP_ObjFusType_FR_Confirm,ObjectType,Object_Dx,Object_Dy,PP_ObjMovingDirSignalProcessing,Object_HeadingAngle,Object_VX,Object_VY,VIE_EgoVelocity,psiDtOpt,axvRefMs2,AEBJunc_Target_ObjectID_K1,AEBJunc_Target_ObjectType_K1
  Bus Selector1 : BusSelector  OutputSignals=Object_ID,PP_ObjFusType_FC_FR_Confirm,PP_ObjFusType_FR_Confirm,ObjectType,Object_Dx,Object_Dy,PP_ObjMovingDirSignalProcessing,Object_HeadingAngle,Object_VX,Object_VY,VIE_EgoVelocity,psiDtOpt,axvRefMs2,AEBJunc_Target_ObjectID_K1,AEBJunc_Target_ObjectType_K1,Object_MovingState
  TOS_AEBJunc_PedTargetsDx : Outport
  TOS_AEBJunc_VehTargetsDx : Outport  Port=2
  AEBJunc_PedTargetFusionType_observal : Outport  Port=3
  AEBJunc_PedTargetObjectType_observal : Outport  Port=4
  AEBJunc_PedTargetDXDY_observal : Outport  Port=5
  AEBJunc_PedTargetMovDir_observal : Outport  Port=6
  AEBJunc_VehTargetFusionType_observal : Outport  Port=7
  AEBJunc_VehTargetObjectType_observal : Outport  Port=8
  AEBJunc_VehTargetDXDY_observal : Outport  Port=9
  AEBJunc_VehTargetMovDir_observal : Outport  Port=10
  AEBJunc_VehTargetMovState_observal : Outport  Port=11
  wires:
  AEBJunc_PedTargetCondition/1(TOS_AEBJunc_PedTargetsDx) -> TOS_AEBJunc_PedTargetsDx/1
  AEBJunc_PedTargetCondition/2(AEBJunc_PedTargetFusionType_observal) -> AEBJunc_PedTargetFusionType_observal/1
  AEBJunc_PedTargetCondition/3(AEBJunc_PedTargetObjectType_observal) -> AEBJunc_PedTargetObjectType_observal/1
  AEBJunc_PedTargetCondition/4(AEBJunc_PedTargetDXDY_observal) -> AEBJunc_PedTargetDXDY_observal/1
  AEBJunc_PedTargetCondition/5(AEBJunc_PedTargetMovDir_observal) -> AEBJunc_PedTargetMovDir_observal/1
  Object_ID/1 -> Bus Creator/1  "Object_ID"
  PP_ObjFusType_FC_FR_Confirm/1 -> Bus Creator/2  "PP_ObjFusType_FC_FR_Confirm"
  PP_ObjFusType_FR_Confirm/1 -> Bus Creator/3  "PP_ObjFusType_FR_Confirm"
  ObjectType/1 -> Bus Creator/4  "ObjectType"
  Object_Dx/1 -> Bus Creator/5  "Object_Dx"
  Object_Dy/1 -> Bus Creator/6  "Object_Dy"
  PP_ObjMovingDirSignalProcessing/1 -> Bus Creator/7  "PP_ObjMovingDirSignalProcessing"
  Object_HeadingAngle/1 -> Bus Creator/8  "Object_HeadingAngle"
  Object_VX/1 -> Bus Creator/9  "Object_VX"
  Object_VY/1 -> Bus Creator/10  "Object_VY"
  VIE_EgoVelocity/1 -> Bus Creator/11  "VIE_EgoVelocity"
  psiDtOpt/1 -> Bus Creator/12  "psiDtOpt"
  axvRefMs2/1 -> Bus Creator/13  "axvRefMs2"
  AEBJunc_Target_ObjectID_K1/1 -> Bus Creator/15  "AEBJunc_Target_ObjectID_K1"
  AEBJunc_Target_ObjectType_K1/1 -> Bus Creator/16  "AEBJunc_Target_ObjectType_K1"
  Bus Creator/1 -> Bus Selector1/1, Bus Selector/1
  Bus Selector/1 -> AEBJunc_PedTargetCondition/1(Object_ID)  "<Object_ID>"
  Bus Selector/2 -> AEBJunc_PedTargetCondition/2(PP_ObjFusType_FC_FR_Confirm)  "<PP_ObjFusType_FC_FR_Confirm>"
  Bus Selector/3 -> AEBJunc_PedTargetCondition/3(PP_ObjFusType_FR_Confirm)  "<PP_ObjFusType_FR_Confirm>"
  Bus Selector/4 -> AEBJunc_PedTargetCondition/4(ObjectType)  "<ObjectType>"
  Bus Selector/5 -> AEBJunc_PedTargetCondition/5(Object_Dx)  "<Object_Dx>"
  Bus Selector/6 -> AEBJunc_PedTargetCondition/6(Object_Dy)  "<Object_Dy>"
  Bus Selector/7 -> AEBJunc_PedTargetCondition/7(PP_ObjMovingDirSignalProcessing)  "<PP_ObjMovingDirSignalProcessing>"
  Bus Selector/8 -> AEBJunc_PedTargetCondition/8(Object_HeadingAngle)  "<Object_HeadingAngle>"
  Bus Selector/9 -> AEBJunc_PedTargetCondition/9(Object_VX)  "<Object_VX>"
  Bus Selector/10 -> AEBJunc_PedTargetCondition/10(Object_VY)  "<Object_VY>"
  Bus Selector/11 -> AEBJunc_PedTargetCondition/11(VIE_EgoVelocity)  "<VIE_EgoVelocity>"
  Bus Selector/12 -> AEBJunc_PedTargetCondition/12(psiDtOpt)  "<psiDtOpt>"
  Bus Selector/13 -> AEBJunc_PedTargetCondition/13(axvRefMs2)  "<axvRefMs2>"
  Bus Selector/14 -> AEBJunc_PedTargetCondition/14(AEBJunc_PedTarget_ObjectID_K1)  "<AEBJunc_Target_ObjectID_K1>"
  Bus Selector/15 -> AEBJunc_PedTargetCondition/15(AEBJunc_Target_ObjectType_K1)  "<AEBJunc_Target_ObjectType_K1>"
  Bus Selector1/15 -> AEBJunc_VehTargetCondition/15(AEBJunc_Target_ObjectType_K1)  "<AEBJunc_Target_ObjectType_K1>"
  Bus Selector1/14 -> AEBJunc_VehTargetCondition/14(AEBJunc_VehTarget_ObjectID_K1)  "<AEBJunc_Target_ObjectID_K1>"
  Bus Selector1/13 -> AEBJunc_VehTargetCondition/13(axvRefMs2)  "<axvRefMs2>"
  Bus Selector1/12 -> AEBJunc_VehTargetCondition/12(psiDtOpt)  "<psiDtOpt>"
  Bus Selector1/11 -> AEBJunc_VehTargetCondition/11(VIE_EgoVelocity)  "<VIE_EgoVelocity>"
  Bus Selector1/10 -> AEBJunc_VehTargetCondition/10(Object_VY)  "<Object_VY>"
  Bus Selector1/9 -> AEBJunc_VehTargetCondition/9(Object_VX)  "<Object_VX>"
  Bus Selector1/8 -> AEBJunc_VehTargetCondition/8(Object_HeadingAngle)  "<Object_HeadingAngle>"
  Bus Selector1/7 -> AEBJunc_VehTargetCondition/7(PP_ObjMovingDirSignalProcessing)  "<PP_ObjMovingDirSignalProcessing>"
  Bus Selector1/6 -> AEBJunc_VehTargetCondition/6(Object_Dy)  "<Object_Dy>"
  Bus Selector1/5 -> AEBJunc_VehTargetCondition/5(Object_Dx)  "<Object_Dx>"
  Bus Selector1/4 -> AEBJunc_VehTargetCondition/4(ObjectType)  "<ObjectType>"
  Bus Selector1/3 -> AEBJunc_VehTargetCondition/3(PP_ObjFusType_FR_Confirm)  "<PP_ObjFusType_FR_Confirm>"
  Bus Selector1/2 -> AEBJunc_VehTargetCondition/2(PP_ObjFusType_FC_FR_Confirm)  "<PP_ObjFusType_FC_FR_Confirm>"
  Bus Selector1/1 -> AEBJunc_VehTargetCondition/1(Object_ID)  "<Object_ID>"
  AEBJunc_VehTargetCondition/5(AEBJunc_VehTargetMovDir_observal) -> AEBJunc_VehTargetMovDir_observal/1
  AEBJunc_VehTargetCondition/4(AEBJunc_VehTargetDXDY_observal) -> AEBJunc_VehTargetDXDY_observal/1
  AEBJunc_VehTargetCondition/3(AEBJunc_VehTargetObjectType_observal) -> AEBJunc_VehTargetObjectType_observal/1
  AEBJunc_VehTargetCondition/2(AEBJunc_VehTargetFusionType_observal) -> AEBJunc_VehTargetFusionType_observal/1
  AEBJunc_VehTargetCondition/1(TOS_AEBJunc_VehTargetsDx) -> TOS_AEBJunc_VehTargetsDx/1
  Object_MovingState/1 -> Bus Creator/14  "Object_MovingState"
  Bus Selector1/16 -> AEBJunc_VehTargetCondition/16(Object_MovingState)  "<Object_MovingState>"
  AEBJunc_VehTargetCondition/6(AEBJunc_VehTargetMovState_observal) -> AEBJunc_VehTargetMovState_observal/1

== system PubIfDecisionTOS_MDL/TOS_20201112/TOS_2012080320/TOS/AEB/TOS_AEBJunct_20201208/AEBJunc_Object_Condition/AEBJA_TargetCondition/TOS_AEBJunc_TargetsConditionDefault ==
  Action Port : ActionPort  ActionPortLabel=if(u1 ~= 0)
  Constant{1,3..5,7..11} (9 alike) : Constant  Value=0  OutDataTypeStr=boolean
  Constant2 : Constant  Value=255  OutDataTypeStr=single
  Constant6 : Constant  Value=255  OutDataTypeStr=single
  TOS_AEBJunc_PedTargetsDx : Outport
  TOS_AEBJunc_VehTargetsDx : Outport  Port=2
  AEBJunc_PedTargetFusionType_observal : Outport  Port=3
  AEBJunc_PedTargetObjectType_observal : Outport  Port=4
  AEBJunc_PedTargetDXDY_observal : Outport  Port=5
  AEBJunc_PedTargetMovDir_observal : Outport  Port=6
  AEBJunc_VehTargetFusionType_observal : Outport  Port=7
  AEBJunc_VehTargetObjectType_observal : Outport  Port=8
  AEBJunc_VehTargetDXDY_observal : Outport  Port=9
  AEBJunc_VehTargetMovDir_observal : Outport  Port=10
  AEBJunc_VehTargetMovState_observal : Outport  Port=11
  wires:
  Constant2/1 -> TOS_AEBJunc_PedTargetsDx/1
  Constant3/1 -> AEBJunc_PedTargetObjectType_observal/1
  Constant1/1 -> AEBJunc_PedTargetFusionType_observal/1
  Constant4/1 -> AEBJunc_PedTargetDXDY_observal/1
  Constant5/1 -> AEBJunc_PedTargetMovDir_observal/1
  Constant6/1 -> TOS_AEBJunc_VehTargetsDx/1
  Constant10/1 -> AEBJunc_VehTargetMovDir_observal/1
  Constant9/1 -> AEBJunc_VehTargetDXDY_observal/1
  Constant7/1 -> AEBJunc_VehTargetFusionType_observal/1
  Constant8/1 -> AEBJunc_VehTargetObjectType_observal/1
  Constant11/1 -> AEBJunc_VehTargetMovState_observal/1
